simulink model "Plant"  (R2023a)
settings: Solver=VariableStepAuto  StartTime=0.0  StopTime=10.0  RelTol=1e-3
undefined symbols (not defined in the file): B_total, c, C, C_alpha_f, C_r, E, e_p0, g, Iz, J_total, l_f, l_r, m, n_st, T_f_total
settings Model: Creator=Tan_Tram  LastModifiedBy=Tan_Tram

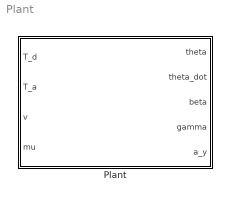
== system Plant ==
  Plant : Subsystem

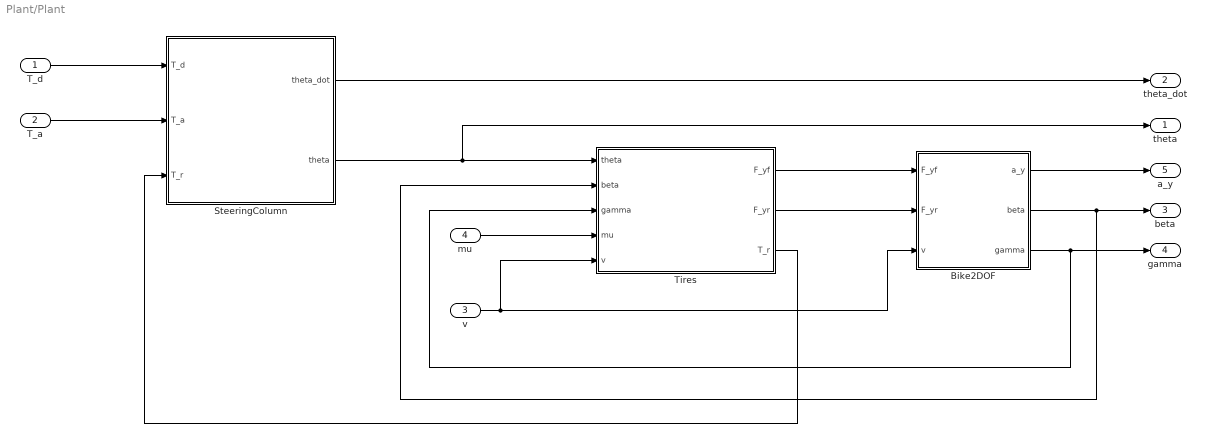
== system Plant/Plant ==
  T_d : Inport
  T_a : Inport  Port=2
  v : Inport  Port=3
  mu : Inport  Port=4
  Bike2DOF : Subsystem
  SteeringColumn : Subsystem
  Tires : Subsystem
  theta : Outport
  theta_dot : Outport  Port=2
  beta : Outport  Port=3
  gamma : Outport  Port=4
  a_y : Outport  Port=5
  wires:
  Bike2DOF/2(beta) -> beta/1, Tires/2(beta)
  T_a/1 -> SteeringColumn/2(T_a)
  T_d/1 -> SteeringColumn/1(T_d)
  mu/1 -> Tires/4(mu)
  v/1 -> Tires/5(v), Bike2DOF/3(v)
  Tires/3(T_r) -> SteeringColumn/3(T_r)
  Tires/2(F_yr) -> Bike2DOF/2(F_yr)
  Tires/1(F_yf) -> Bike2DOF/1(F_yf)
  Bike2DOF/3(gamma) -> gamma/1, Tires/3(gamma)
  Bike2DOF/1(a_y) -> a_y/1
  SteeringColumn/2(theta) -> theta/1, Tires/1(theta)
  SteeringColumn/1(theta_dot) -> theta_dot/1

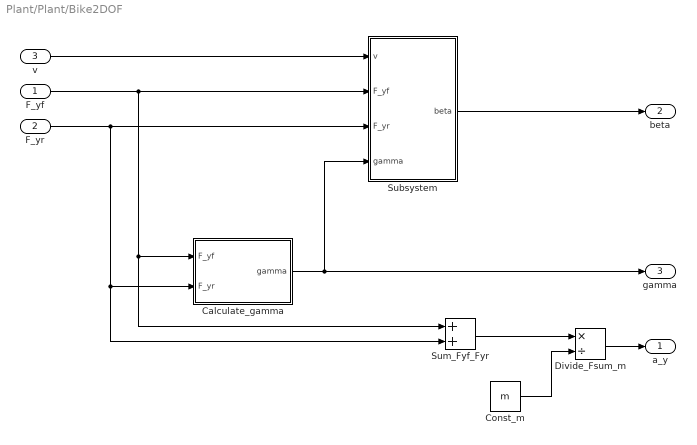
== system Plant/Plant/Bike2DOF ==
  F_yf : Inport
  F_yr : Inport  Port=2
  v : Inport  Port=3
  Calculate_gamma : Subsystem
  Const_m : Constant  Value=m
  Divide_Fsum_m : Product  Inputs=*/
  Subsystem : Subsystem
  Sum_Fyf_Fyr : Sum
  a_y : Outport
  beta : Outport  Port=2
  gamma : Outport  Port=3
  wires:
  Subsystem/1(beta) -> beta/1
  v/1 -> Subsystem/1(v)
  Calculate_gamma/1(gamma) -> gamma/1, Subsystem/4(gamma)
  Divide_Fsum_m/1 -> a_y/1
  Sum_Fyf_Fyr/1 -> Divide_Fsum_m/1
  Const_m/1 -> Divide_Fsum_m/2
  F_yr/1 -> Subsystem/3(F_yr), Sum_Fyf_Fyr/2, Calculate_gamma/2(F_yr)
  F_yf/1 -> Sum_Fyf_Fyr/1, Calculate_gamma/1(F_yf), Subsystem/2(F_yf)

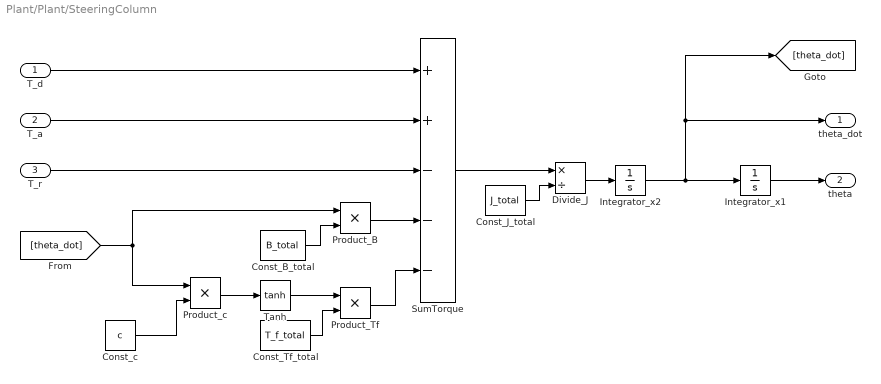
== system Plant/Plant/SteeringColumn ==
  T_d : Inport
  T_a : Inport  Port=2
  T_r : Inport  Port=3
  Const_B_total : Constant  Value=B_total
  Const_J_total : Constant  Value=J_total
  Const_Tf_total : Constant  Value=T_f_total
  Const_c : Constant  Value=c
  Divide_J : Product  Inputs=*/
  Integrator_x1 : Integrator
  Integrator_x2 : Integrator
  Product_B : Product
  Product_Tf : Product
  Product_c : Product
  SumTorque : Sum  Inputs=++---
  Tanh : Trigonometry  Operator=tanh
  theta_dot : Outport
  theta : Outport  Port=2
  wires:
  [theta_dot] -> Product_B/1, Product_c/1
  Integrator_x1/1 -> theta/1
  Divide_J/1 -> Integrator_x2/1
  Const_J_total/1 -> Divide_J/2
  SumTorque/1 -> Divide_J/1
  Product_Tf/1 -> SumTorque/5
  Const_Tf_total/1 -> Product_Tf/2
  Tanh/1 -> Product_Tf/1
  Product_c/1 -> Tanh/1
  Const_c/1 -> Product_c/2
  Product_B/1 -> SumTorque/4
  Const_B_total/1 -> Product_B/2
  Integrator_x2/1 -> theta_dot/1, [theta_dot], Integrator_x1/1
  T_r/1 -> SumTorque/3
  T_a/1 -> SumTorque/2
  T_d/1 -> SumTorque/1

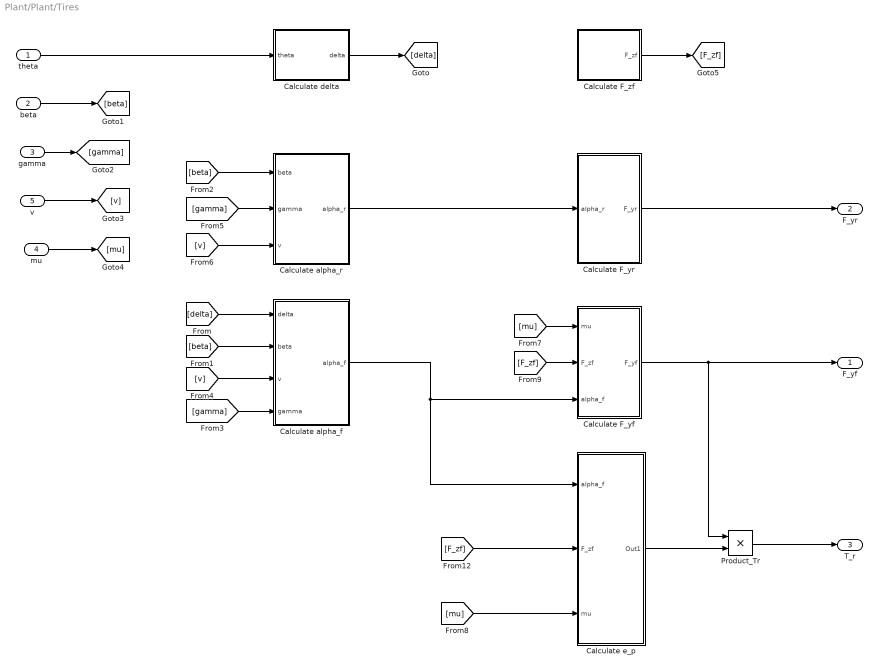
== system Plant/Plant/Tires ==
  theta : Inport
  beta : Inport  Port=2
  gamma : Inport  Port=3
  mu : Inport  Port=4
  v : Inport  Port=5
  Calculate F_yf : Subsystem
  Calculate F_yr : Subsystem
  Calculate F_zf : Subsystem
  Calculate alpha_f : Subsystem
  Calculate alpha_r : Subsystem
  Calculate delta : Subsystem
  Calculate e_p : Subsystem
  Product_Tr : Product  Inputs=**
  F_yf : Outport
  F_yr : Outport  Port=2
  T_r : Outport  Port=3
  wires:
  Calculate e_p/1(Out1) -> Product_Tr/2
  [mu] -> Calculate e_p/3(mu)
  [F_zf] -> Calculate e_p/2(F_zf)
  Calculate alpha_f/1(alpha_f) -> Calculate e_p/1(alpha_f), Calculate F_yf/3(alpha_f)
  Calculate F_yr/1(F_yr) -> F_yr/1
  Calculate alpha_r/1(alpha_r) -> Calculate F_yr/1(alpha_r)
  [F_zf] -> Calculate F_yf/2(F_zf)
  [mu] -> Calculate F_yf/1(mu)
  Calculate F_yf/1(F_yf) -> Product_Tr/1, F_yf/1
  Calculate F_zf/1(F_zf) -> [F_zf]
  mu/1 -> [mu]
  [v] -> Calculate alpha_r/3(v)
  [gamma] -> Calculate alpha_r/2(gamma)
  [beta] -> Calculate alpha_r/1(beta)
  [v] -> Calculate alpha_f/3(v)
  v/1 -> [v]
  [gamma] -> Calculate alpha_f/4(gamma)
  gamma/1 -> [gamma]
  [beta] -> Calculate alpha_f/2(beta)
  beta/1 -> [beta]
  Calculate delta/1(delta) -> [delta]
  [delta] -> Calculate alpha_f/1(delta)
  theta/1 -> Calculate delta/1(theta)
  Product_Tr/1 -> T_r/1

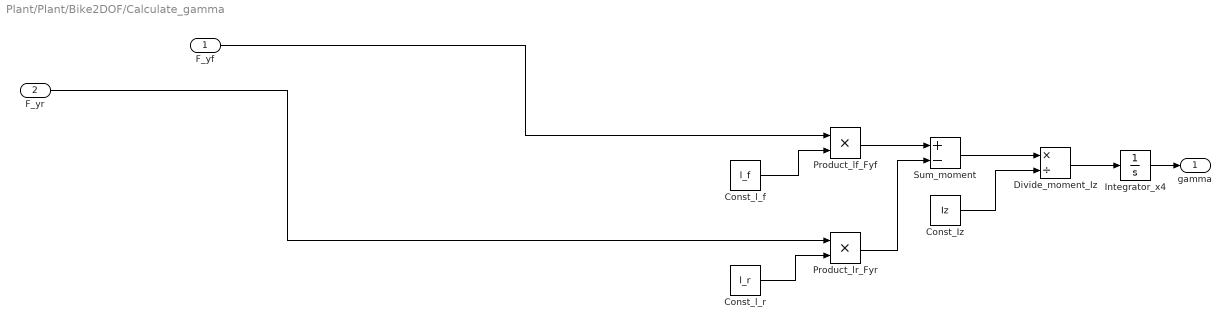
== system Plant/Plant/Bike2DOF/Calculate_gamma ==
  F_yf : Inport
  F_yr : Inport  Port=2
  Const_Iz : Constant  Value=Iz
  Const_l_f : Constant  Value=l_f
  Const_l_r : Constant  Value=l_r
  Divide_moment_Iz : Product  Inputs=*/
  Integrator_x4 : Integrator
  Product_lf_Fyf : Product  Inputs=**
  Product_lr_Fyr : Product  Inputs=**
  Sum_moment : Sum  Inputs=+-
  gamma : Outport
  wires:
  F_yr/1 -> Product_lr_Fyr/1
  F_yf/1 -> Product_lf_Fyf/1
  Product_lr_Fyr/1 -> Sum_moment/2
  Const_l_f/1 -> Product_lf_Fyf/2
  Sum_moment/1 -> Divide_moment_Iz/1
  Const_Iz/1 -> Divide_moment_Iz/2
  Integrator_x4/1 -> gamma/1
  Divide_moment_Iz/1 -> Integrator_x4/1
  Product_lf_Fyf/1 -> Sum_moment/1
  Const_l_r/1 -> Product_lr_Fyr/2

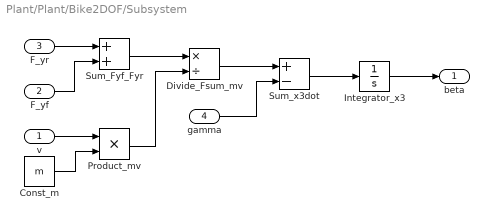
== system Plant/Plant/Bike2DOF/Subsystem ==
  v : Inport
  F_yf : Inport  Port=2
  F_yr : Inport  Port=3
  gamma : Inport  Port=4
  Const_m : Constant  Value=m
  Divide_Fsum_mv : Product  Inputs=*/
  Integrator_x3 : Integrator
  Product_mv : Product  Inputs=**
  Sum_Fyf_Fyr : Sum
  Sum_x3dot : Sum  Inputs=+-
  beta : Outport
  wires:
  Integrator_x3/1 -> beta/1
  Sum_x3dot/1 -> Integrator_x3/1
  Divide_Fsum_mv/1 -> Sum_x3dot/1
  v/1 -> Product_mv/1
  Const_m/1 -> Product_mv/2
  gamma/1 -> Sum_x3dot/2
  F_yr/1 -> Sum_Fyf_Fyr/1
  F_yf/1 -> Sum_Fyf_Fyr/2
  Sum_Fyf_Fyr/1 -> Divide_Fsum_mv/1
  Product_mv/1 -> Divide_Fsum_mv/2

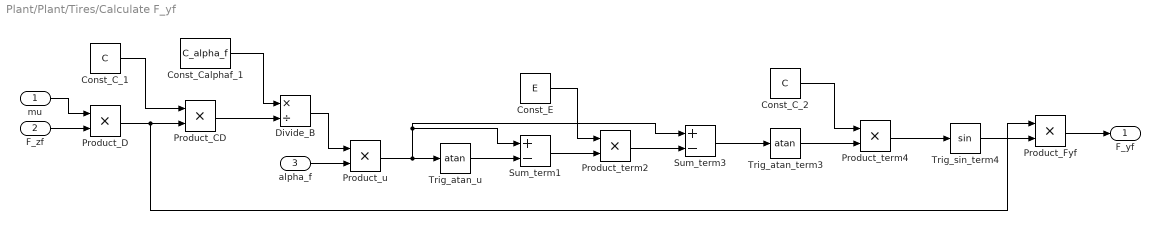
== system Plant/Plant/Tires/Calculate F_yf ==
  mu : Inport
  F_zf : Inport  Port=2
  alpha_f : Inport  Port=3
  Const_C_1 : Constant  Value=C
  Const_C_2 : Constant  Value=C
  Const_Calphaf_1 : Constant  Value=C_alpha_f
  Const_E : Constant  Value=E
  Divide_B : Product  Inputs=*/
  Product_CD : Product  Inputs=**
  Product_D : Product  Inputs=**
  Product_Fyf : Product  Inputs=**
  Product_term2 : Product  Inputs=**
  Product_term4 : Product  Inputs=**
  Product_u : Product  Inputs=**
  Sum_term1 : Sum  Inputs=+-
  Sum_term3 : Sum  Inputs=+-
  Trig_atan_term3 : Trigonometry  Operator=atan
  Trig_atan_u : Trigonometry  Operator=atan
  Trig_sin_term4 : Trigonometry
  F_yf : Outport
  wires:
  Product_Fyf/1 -> F_yf/1
  Trig_sin_term4/1 -> Product_Fyf/2
  Product_term4/1 -> Trig_sin_term4/1
  Trig_atan_term3/1 -> Product_term4/2
  Const_C_2/1 -> Product_term4/1
  Product_term2/1 -> Sum_term3/2
  Trig_atan_u/1 -> Sum_term1/2
  Product_u/1 -> Trig_atan_u/1, Sum_term1/1, Sum_term3/1
  Sum_term3/1 -> Trig_atan_term3/1
  Product_D/1 -> Product_Fyf/1, Product_CD/2
  Product_CD/1 -> Divide_B/2
  Const_C_1/1 -> Product_CD/1
  Const_E/1 -> Product_term2/1
  Const_Calphaf_1/1 -> Divide_B/1
  mu/1 -> Product_D/1
  F_zf/1 -> Product_D/2
  Divide_B/1 -> Product_u/1
  Sum_term1/1 -> Product_term2/2
  alpha_f/1 -> Product_u/2

== system Plant/Plant/Tires/Calculate F_yr ==
  alpha_r : Inport
  Const_C_r : Constant  Value=C_r
  Product_Fyr : Product  Inputs=**
  F_yr : Outport
  wires:
  Product_Fyr/1 -> F_yr/1
  alpha_r/1 -> Product_Fyr/2
  Const_C_r/1 -> Product_Fyr/1

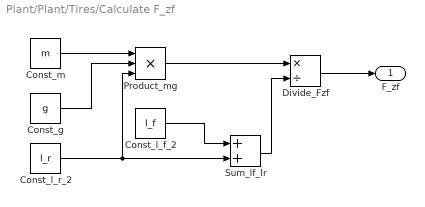
== system Plant/Plant/Tires/Calculate F_zf ==
  Const_g : Constant  Value=g
  Const_l_f_2 : Constant  Value=l_f
  Const_l_r_2 : Constant  Value=l_r
  Const_m : Constant  Value=m
  Divide_Fzf : Product  Inputs=*/
  Product_mg : Product  Inputs=***
  Sum_lf_lr : Sum
  F_zf : Outport
  wires:
  Const_l_f_2/1 -> Sum_lf_lr/1
  Sum_lf_lr/1 -> Divide_Fzf/2
  Const_g/1 -> Product_mg/2
  Const_m/1 -> Product_mg/1
  Product_mg/1 -> Divide_Fzf/1
  Divide_Fzf/1 -> F_zf/1
  Const_l_r_2/1 -> Product_mg/3, Sum_lf_lr/2

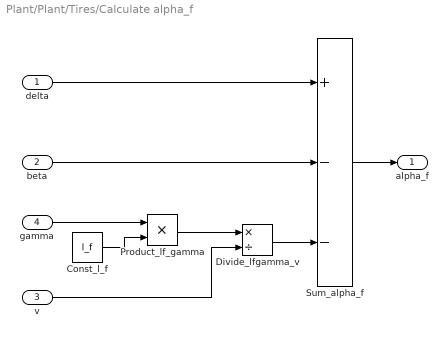
== system Plant/Plant/Tires/Calculate alpha_f ==
  delta : Inport
  beta : Inport  Port=2
  v : Inport  Port=3
  gamma : Inport  Port=4
  Const_l_f : Constant  Value=l_f
  Divide_lfgamma_v : Product  Inputs=*/
  Product_lf_gamma : Product  Inputs=**
  Sum_alpha_f : Sum  Inputs=+--
  alpha_f : Outport
  wires:
  Const_l_f/1 -> Product_lf_gamma/2
  Sum_alpha_f/1 -> alpha_f/1
  Divide_lfgamma_v/1 -> Sum_alpha_f/3
  Product_lf_gamma/1 -> Divide_lfgamma_v/1
  gamma/1 -> Product_lf_gamma/1
  v/1 -> Divide_lfgamma_v/2
  beta/1 -> Sum_alpha_f/2
  delta/1 -> Sum_alpha_f/1

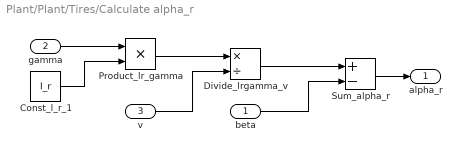
== system Plant/Plant/Tires/Calculate alpha_r ==
  beta : Inport
  gamma : Inport  Port=2
  v : Inport  Port=3
  Const_l_r_1 : Constant  Value=l_r
  Divide_lrgamma_v : Product  Inputs=*/
  Product_lr_gamma : Product  Inputs=**
  Sum_alpha_r : Sum  Inputs=+-
  alpha_r : Outport
  wires:
  Divide_lrgamma_v/1 -> Sum_alpha_r/1
  beta/1 -> Sum_alpha_r/2
  Sum_alpha_r/1 -> alpha_r/1
  v/1 -> Divide_lrgamma_v/2
  Product_lr_gamma/1 -> Divide_lrgamma_v/1
  Const_l_r_1/1 -> Product_lr_gamma/2
  gamma/1 -> Product_lr_gamma/1

== system Plant/Plant/Tires/Calculate delta ==
  theta : Inport
  Const_n_st : Constant  Value=n_st
  Divide_delta : Product  Inputs=*/
  delta : Outport
  wires:
  Const_n_st/1 -> Divide_delta/2
  Divide_delta/1 -> delta/1
  theta/1 -> Divide_delta/1

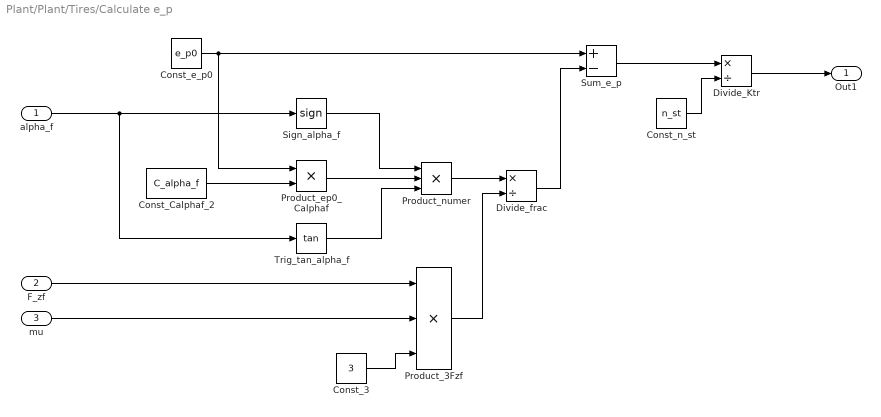
== system Plant/Plant/Tires/Calculate e_p ==
  alpha_f : Inport
  F_zf : Inport  Port=2
  mu : Inport  Port=3
  Const_3 : Constant  Value=3
  Const_Calphaf_2 : Constant  Value=C_alpha_f
  Const_e_p0 : Constant  Value=e_p0
  Const_n_st : Constant  Value=n_st
  Divide_Ktr : Product  Inputs=*/
  Divide_frac : Product  Inputs=*/
  Product_3Fzf : Product  Inputs=***
  Product_ep0_Calphaf : Product  Inputs=**
  Product_numer : Product  Inputs=***
  Sign_alpha_f : Signum
  Sum_e_p : Sum  Inputs=+-
  Trig_tan_alpha_f : Trigonometry  Operator=tan
  Out1 : Outport
  wires:
  F_zf/1 -> Product_3Fzf/1
  Divide_Ktr/1 -> Out1/1
  Product_3Fzf/1 -> Divide_frac/2
  Const_3/1 -> Product_3Fzf/3
  Const_n_st/1 -> Divide_Ktr/2
  Const_Calphaf_2/1 -> Product_ep0_Calphaf/2
  Divide_frac/1 -> Sum_e_p/2
  mu/1 -> Product_3Fzf/2
  Const_e_p0/1 -> Product_ep0_Calphaf/1, Sum_e_p/1
  Product_numer/1 -> Divide_frac/1
  Product_ep0_Calphaf/1 -> Product_numer/2
  Sign_alpha_f/1 -> Product_numer/1
  alpha_f/1 -> Sign_alpha_f/1, Trig_tan_alpha_f/1
  Trig_tan_alpha_f/1 -> Product_numer/3
  Sum_e_p/1 -> Divide_Ktr/1
